simulink model "battery_sim"  (R2025b)
settings: Solver=VariableStepAuto  StartTime=0.0  StopTime=10.0  RelTol=1e-3
values from neighbouring files (symbols this model uses):
  C1_pack = C1_cell * N_parallel / N_series    (= 846.153846154)    [battery_parameters.m]
  load_current = 10    [battery_parameters.m]
  OCV_pack = OCV_cell * N_series    [battery_parameters.m]
  Q_pack = Q_cell * N_parallel    (= 35.2)    [battery_parameters.m]
  R1_pack = R1_cell / N_parallel * N_series    (= 0.00590909090909)    [battery_parameters.m]
  Rs_pack = Rs_cell / N_parallel * N_series    (= 0.0177272727273)    [battery_parameters.m]
  SOC_initial = 1.0    (= 1)    [battery_parameters.m]
  SOC_lookup = [0.0  0.1  0.2  0.3  0.4  0.5  0.6  0.7  0.8  0.9  1.0]    [battery_parameters.m]

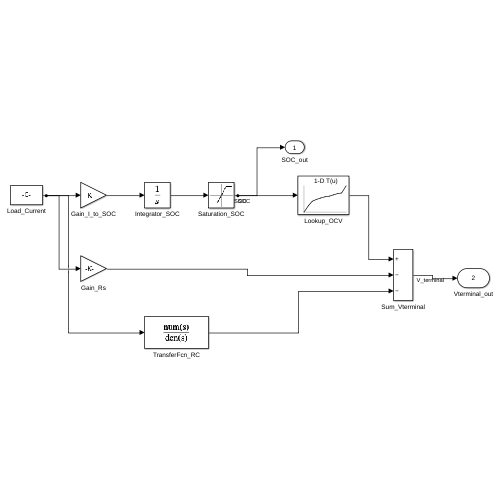
[thumbnail: Simulink's stored preview of the top-level diagram]
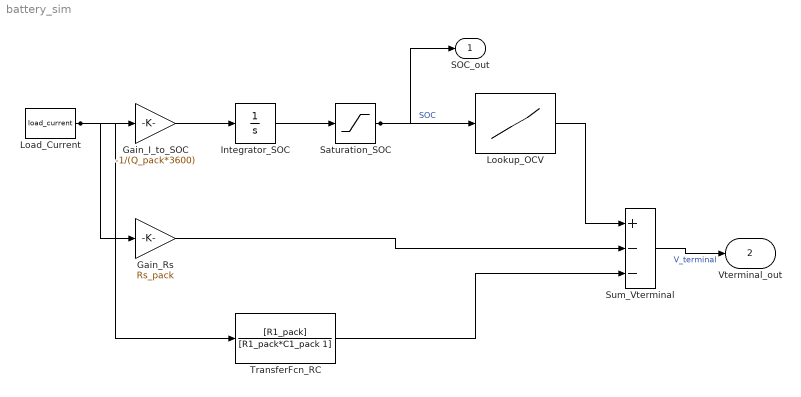
== system battery_sim ==
  Gain_I_to_SOC : Gain  Gain=-1/(Q_pack*3600)
  Gain_Rs : Gain  Gain=Rs_pack
  Integrator_SOC : Integrator  InitialCondition=SOC_initial
  Load_Current : Constant  Value=load_current
  Lookup_OCV : Lookup_n-D  NumberOfTableDimensions=1  BreakpointsForDimension1=SOC_lookup  Table=OCV_pack  InternalRulePriority=Speed  RndMeth=Simplest
  Saturation_SOC : Saturate  UpperLimit=1  LowerLimit=0
  Sum_Vterminal : Sum  Inputs=+--
  TransferFcn_RC : TransferFcn  Numerator=[R1_pack]  Denominator=[R1_pack*C1_pack 1]
  SOC_out : Outport
  Vterminal_out : Outport  Port=2
  wires:
  Load_Current/1 -> Gain_I_to_SOC/1, Gain_Rs/1, TransferFcn_RC/1
  Gain_I_to_SOC/1 -> Integrator_SOC/1
  Integrator_SOC/1 -> Saturation_SOC/1
  Saturation_SOC/1 -> Lookup_OCV/1, SOC_out/1  "SOC"
  Lookup_OCV/1 -> Sum_Vterminal/1
  Gain_Rs/1 -> Sum_Vterminal/2
  TransferFcn_RC/1 -> Sum_Vterminal/3
  Sum_Vterminal/1 -> Vterminal_out/1  "V_terminal"
